simulink model "q_heli_2d_open_loop"  (Simulink 8.8)
settings: Solver=FixedStepAuto  StartTime=0.0  StopTime=10  FixedStep=1e-3  RelTol=1e-3
values from neighbouring files (symbols this model uses):
  K_AMP = 1    [setup_lab_heli_2d.m]
  K_EC_P = 2 * pi / 2400    (= 0.00261799387799)    [setup_lab_heli_2d.m]
  K_EC_Y = 2 * pi / 2400    (= 0.00261799387799)    [setup_lab_heli_2d.m]
  theta_0 = -47*pi/180    (= -0.820304748437)    [setup_lab_heli_2d.m]
  VMAX_AMP_P = 3.2    [setup_lab_heli_2d.m]
  VMAX_AMP_Y = 3.2    [setup_lab_heli_2d.m]
  wcf = 2 * pi * 20    (= 125.663706144)    [setup_lab_heli_2d.m]
  zetaf = 0.85    [setup_lab_heli_2d.m]
undefined symbols (not defined in the file or in its folder): MultiQ, PCI, Quanser
libraries: sldrtlib x4, simulink_extras x3
settings Model: Creator=MLevis  LastModifiedBy=Labos1  SimulationMode=external  ExtModeTrigDuration=50000
settings OptimizationCC: BooleanDataType=off  OptimizeBlockIOStorage=off  BufferReuse=off  GlobalBufferReuse=off  ExpressionFolding=off  ExpressionDepthLimit=2147483647  LocalBlockOutputs=off  InitFltsAndDblsToZero=on  LifeSpan=auto
settings DebuggingCC: SaveWithParameterizedLinksMsg=none  SignalResolutionControl=TryResolveAllWithWarning  SolverPrmCheckMsg=warning  MultiTaskDSMMsg=warning  MultiTaskCondExecSysMsg=none
settings HardwareCC: ProdBitPerPointer=64  ProdBitPerSizeT=64  ProdBitPerPtrDiffT=64  ProdLargestAtomicFloat=Float  ProdIntDivRoundTo=Zero  ProdEndianess=LittleEndian  ProdWordSize=64  ProdHWDeviceType=Intel->x86-64 (Windows64)
settings RTWCC: SystemTargetFile=sldrt.tlc  TemplateMakefile=sldrt.tmf  Description=Simulink Desktop Real-Time  RTWCompilerOptimization=on
settings CodeAppCC: MaxIdLength=95
settings SimulinkDesktopRealTimeCC: TargetPreCompLibLocation=C:\Program Files\MATLAB\R2016b\toolbox\sldrt\lib\win64  TargetLangStandard=C89/C90 (ANSI)  SupportVariableSizeSignals=off

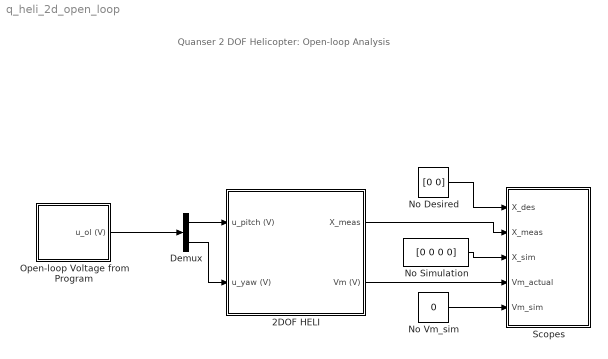
== system q_heli_2d_open_loop ==
  note: Quanser 2 DOF Helicopter:
      | Open-loop Analysis
  2DOF HELI : Subsystem
  Demux : Demux  Outputs=2
  No Desired : Constant  Value=[0 0]
  No Simulation : Constant  Value=[0 0 0 0]
  No Vm_sim : Constant  Value=0
  Open-loop Voltage from Program : Subsystem
  Scopes : Subsystem
  wires:
  Open-loop Voltage from Program/1(u_ol (V)) -> Demux/1
  Demux/1 -> 2DOF HELI/1(u_pitch (V))
  Demux/2 -> 2DOF HELI/2(u_yaw (V))
  2DOF HELI/1(X_meas) -> Scopes/2(X_meas)
  2DOF HELI/2(Vm (V)) -> Scopes/4(Vm_actual)
  No Desired/1 -> Scopes/1(X_des)
  No Simulation/1 -> Scopes/3(X_sim)
  No Vm_sim/1 -> Scopes/5(Vm_sim)

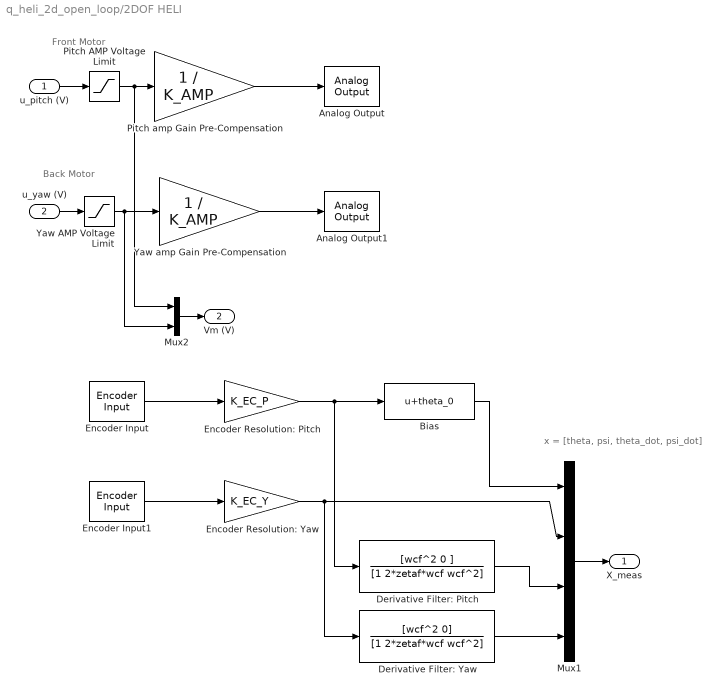
== system q_heli_2d_open_loop/2DOF HELI ==
  note: Back Motor
  note: Front Motor
  note: x = [theta, psi, theta_dot, psi_dot]
  u_pitch (V) : Inport
  u_yaw (V) : Inport  Port=2
  Analog Output : sldrtlib/Analog Output  SampleTime=1e-3  MaxMissedTicks=10  ShowMissedTicks=off  YieldWhenWaiting=off  DrvName=Quanser/MultiQ-PCI  DrvAddress=4294967295  DrvOptions=zeros(1,0)  Channels=1  RangeMode=1  VoltRange=1  InitialValue=0  FinalValue=0
      settings: AttributesFormatString=Quanser\nMultiQ-PCI [auto]
  Analog Output1 : sldrtlib/Analog Output  SampleTime=1e-3  MaxMissedTicks=10  ShowMissedTicks=off  YieldWhenWaiting=off  DrvName=Quanser/MultiQ-PCI  DrvAddress=4294967295  DrvOptions=zeros(1,0)  Channels=2  RangeMode=1  VoltRange=1  InitialValue=0  FinalValue=0
      settings: AttributesFormatString=Quanser\nMultiQ-PCI [auto]
  Bias : Bias  Bias=theta_0
  Derivative Filter: Pitch : TransferFcn  Numerator=[wcf^2 0 ]  Denominator=[1 2*zetaf*wcf wcf^2]
  Derivative Filter: Yaw : TransferFcn  Numerator=[wcf^2 0]  Denominator=[1 2*zetaf*wcf wcf^2]
  Encoder Input : sldrtlib/Encoder Input  SampleTime=1e-3  MaxMissedTicks=10  ShowMissedTicks=off  YieldWhenWaiting=off  DrvName=Quanser/MultiQ-PCI  DrvAddress=4294967295  DrvOptions=zeros(1,0)  Channels=1  QuadMode=3  IndexPulse=2  InputFilter=Inf  DataType=1
      settings: AttributesFormatString=Quanser\nMultiQ-PCI [auto]
  Encoder Input1 : sldrtlib/Encoder Input  SampleTime=1e-3  MaxMissedTicks=10  ShowMissedTicks=off  YieldWhenWaiting=off  DrvName=Quanser/MultiQ-PCI  DrvAddress=4294967295  DrvOptions=zeros(1,0)  Channels=2  QuadMode=3  IndexPulse=2  InputFilter=Inf  DataType=1
      settings: AttributesFormatString=Quanser\nMultiQ-PCI [auto]
  "Encoder Resolution: Pitch " : Gain  Gain=K_EC_P
  Encoder Resolution: Yaw : Gain  Gain=K_EC_Y
  Mux1 : Mux
  Mux2 : Mux  Inputs=2
  Pitch AMP Voltage Limit : Saturate  UpperLimit=VMAX_AMP_P  LowerLimit=- VMAX_AMP_P
  Pitch amp Gain Pre-Compensation : Gain  Gain=1 / K_AMP  SaturateOnIntegerOverflow=on  OutDataTypeStr=Inherit: Same as input  ParamDataTypeStr=Inherit: Same as input
  Yaw AMP Voltage Limit : Saturate  UpperLimit=VMAX_AMP_Y  LowerLimit=- VMAX_AMP_Y
  Yaw amp Gain Pre-Compensation : Gain  Gain=1 / K_AMP  SaturateOnIntegerOverflow=on  OutDataTypeStr=Inherit: Same as input  ParamDataTypeStr=Inherit: Same as input
  X_meas : Outport
  Vm (V) : Outport  Port=2
  wires:
  Encoder Resolution: Yaw/1 -> Mux1/2, Derivative Filter: Yaw/1
  Mux2/1 -> Vm (V)/1
  Yaw amp Gain Pre-Compensation/1 -> Analog Output1/1
  Pitch amp Gain Pre-Compensation/1 -> Analog Output/1
  Mux1/1 -> X_meas/1
  u_yaw (V)/1 -> Yaw AMP Voltage Limit/1
  u_pitch (V)/1 -> Pitch AMP Voltage Limit/1
  Yaw AMP Voltage Limit/1 -> Mux2/2, Yaw amp Gain Pre-Compensation/1
  Pitch AMP Voltage Limit/1 -> Mux2/1, Pitch amp Gain Pre-Compensation/1
  Encoder Input/1 -> "Encoder Resolution: Pitch "/1
  "Encoder Resolution: Pitch "/1 -> Bias/1, Derivative Filter: Pitch/1
  Encoder Input1/1 -> Encoder Resolution: Yaw/1
  Bias/1 -> Mux1/1
  Derivative Filter: Pitch/1 -> Mux1/3
  Derivative Filter: Yaw/1 -> Mux1/4

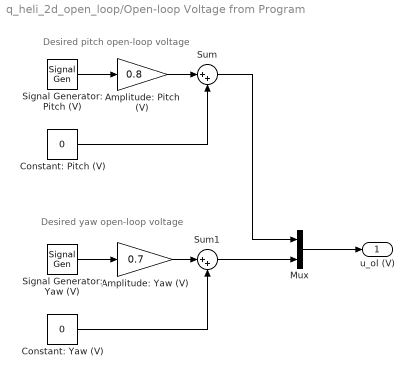
== system q_heli_2d_open_loop/Open-loop Voltage from Program ==
  note: Desired yaw open-loop voltage
  note: Desired pitch open-loop voltage
  Amplitude: Pitch (V) : Gain  Gain=0.8
  Amplitude: Yaw (V) : Gain  Gain=0.7
  Constant: Pitch (V) : Constant  Value=0
  Constant: Yaw (V) : Constant  Value=0
  Mux : Mux  Inputs=2
  Signal Generator: Pitch (V) : SignalGenerator  WaveForm=square  Amplitude=3  Frequency=0.0001
  Signal Generator: Yaw (V) : SignalGenerator  WaveForm=square  Amplitude=3  Frequency=0.4
  Sum : Sum  Inputs=|++
  Sum1 : Sum  Inputs=|++
  u_ol (V) : Outport
  wires:
  Mux/1 -> u_ol (V)/1
  Sum1/1 -> Mux/2
  Sum/1 -> Mux/1
  Signal Generator: Yaw (V)/1 -> Amplitude: Yaw (V)/1
  Amplitude: Yaw (V)/1 -> Sum1/1
  Constant: Yaw (V)/1 -> Sum1/2
  Signal Generator: Pitch (V)/1 -> Amplitude: Pitch (V)/1
  Amplitude: Pitch (V)/1 -> Sum/1
  Constant: Pitch (V)/1 -> Sum/2

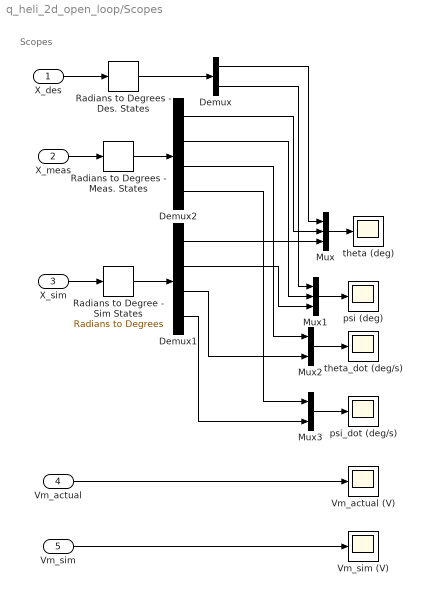
== system q_heli_2d_open_loop/Scopes ==
  note: Scopes
  X_des : Inport
  X_meas : Inport  Port=2
  X_sim : Inport  Port=3
  Vm_actual : Inport  Port=4
  Vm_sim : Inport  Port=5
  Demux : Demux  Outputs=2
  Demux1 : Demux
  Demux2 : Demux
  Mux : Mux  Inputs=3
  Mux1 : Mux  Inputs=3
  Mux2 : Mux  Inputs=2
  Mux3 : Mux  Inputs=2
  Radians to Degree - Sim States : simulink_extras/Transformations/Radians to Degrees
  Radians to Degrees - Des. States : simulink_extras/Transformations/Radians to Degrees
  Radians to Degrees - Meas. States : simulink_extras/Transformations/Radians to Degrees
  Vm_actual (V) : Scope
  Vm_sim (V) : Scope
  psi (deg) : Scope
  psi_dot (deg/s) : Scope
  theta (deg) : Scope
  theta_dot (deg/s) : Scope
  wires:
  Vm_sim/1 -> Vm_sim (V)/1
  Radians to Degrees - Des. States/1 -> Demux/1
  Demux1/2 -> Mux1/3
  Demux2/2 -> Mux1/2
  Demux/2 -> Mux1/1
  Demux1/1 -> Mux/3
  Demux2/1 -> Mux/2
  Demux/1 -> Mux/1
  X_des/1 -> Radians to Degrees - Des. States/1
  Demux2/3 -> Mux2/1
  Demux2/4 -> Mux3/1
  X_meas/1 -> Radians to Degrees - Meas. States/1
  Radians to Degrees - Meas. States/1 -> Demux2/1
  X_sim/1 -> Radians to Degree - Sim States/1
  Radians to Degree - Sim States/1 -> Demux1/1
  Mux/1 -> theta (deg)/1
  Mux1/1 -> psi (deg)/1
  Mux2/1 -> theta_dot (deg/s)/1
  Mux3/1 -> psi_dot (deg/s)/1
  Demux1/3 -> Mux2/2
  Demux1/4 -> Mux3/2
  Vm_actual/1 -> Vm_actual (V)/1
